simulink model "unityfeedback_comparing"  (R2023b)
settings: Solver=VariableStepAuto  StartTime=0.0  StopTime=10.0  RelTol=1e-3
settings Model: Creator=reemb  LastModifiedBy=reemb

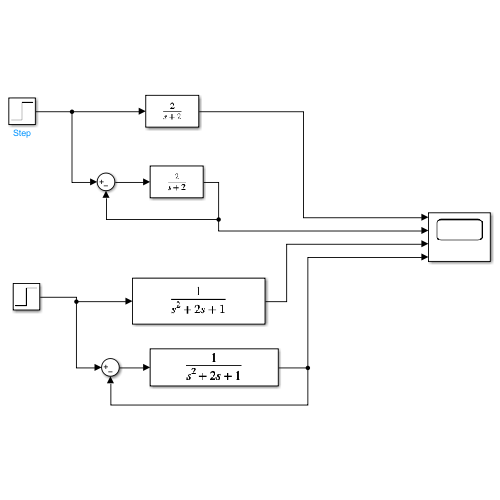
[thumbnail: Simulink's stored preview of the top-level diagram]
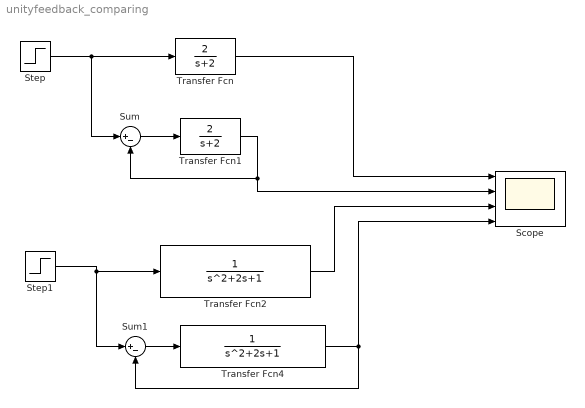
== system unityfeedback_comparing ==
  Scope : Scope  NumInputPorts=4
  Step : Step  SampleTime=0
  Step1 : Step  SampleTime=0
  Sum : Sum  Inputs=|+-
  Sum1 : Sum  Inputs=|+-
  Transfer Fcn : TransferFcn  Numerator=[2]  Denominator=[1 2]
  Transfer Fcn1 : TransferFcn  Numerator=[2]  Denominator=[1 2]
  Transfer Fcn2 : TransferFcn
  Transfer Fcn4 : TransferFcn
  wires:
  Transfer Fcn/1 -> Scope/1
  Step/1 -> Sum/1, Transfer Fcn/1
  Sum/1 -> Transfer Fcn1/1
  Transfer Fcn1/1 -> Scope/2, Sum/2
  Transfer Fcn4/1 -> Scope/4, Sum1/2
  Sum1/1 -> Transfer Fcn4/1
  Step1/1 -> Sum1/1, Transfer Fcn2/1
  Transfer Fcn2/1 -> Scope/3
